simulink model "towTest"  (R2020a)
settings: Solver=FixedStepAuto  StartTime=0.0  StopTime=inf  RelTol=1e-3  EnableMultiTasking=on
undefined symbols (not defined in the file or in its folder): IO397
libraries: slrtlib x5, speedgoatlib_fpga_quadrature x2, dspsigops x2, speedgoatlib_fpga_dio x1, speedgoatlib_fpga_analog_io x1, dspfdesign x1, speedgoatlib_fpga x1, powerlib_meascontrol x1
settings Model: SimulationMode=external  Creator=MAE-VermillionLab  LastModifiedBy=ViconLab
settings SolverCC: ConcurrentTasks=on  AutoInsertRateTranBlk=on
settings DataIOCC: SaveFormat=StructureWithTime
settings OptimizationCC: BlockReduction=off  OptimizeBlockIOStorage=off
settings HardwareCC: ProdBitPerPointer=32  ProdBitPerSizeT=32  ProdBitPerPtrDiffT=32  ProdLargestAtomicFloat=None  ProdWordSize=32  ProdLongLongMode=on  ProdHWDeviceType=Generic->32-bit x86 compatible
settings RTWCC: Description=Simulink Real-Time  SystemTargetFile=slrt.tlc  TemplateMakefile=slrt_default_tmf  CodeExecutionProfiling=on  RTWCompilerOptimization=on
settings SimulinkRealTimeCC: SupportVariableSizeSignals=on  RL32LogTETModifier=off  xPCConcurrentTasks=on

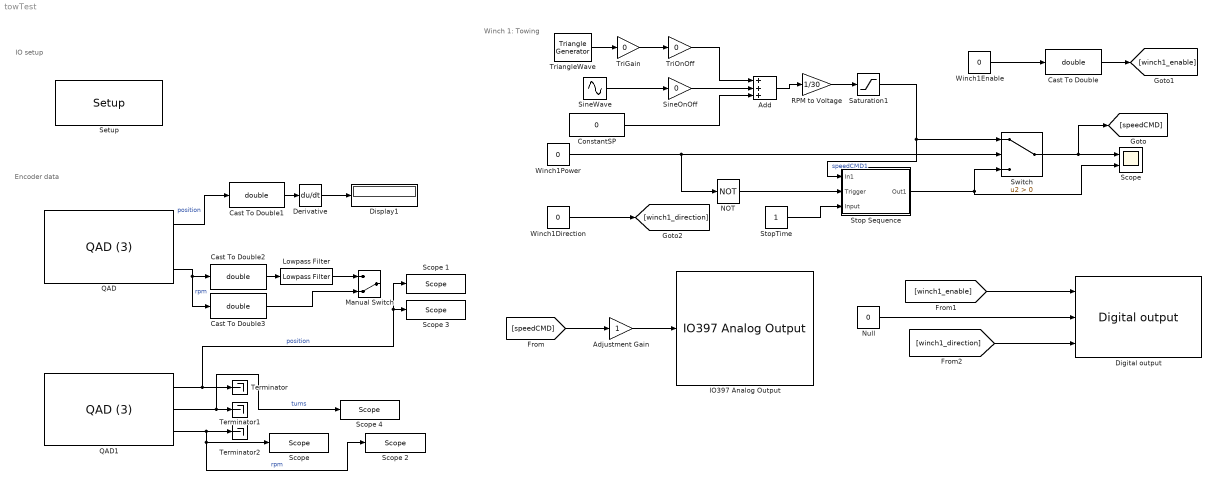
== system towTest ==
  note: Winch 1: Towing
  note: Encoder data
  note: IO setup
  Add : Sum  Inputs=+++
  Adjustment Gain : Gain
  Cast To Double{,1..3} (4 alike) : DataTypeConversion  OutDataTypeStr=double
  ConstantSP : Constant  Value=0
  Derivative : Derivative
  Digital output : speedgoatlib_fpga_dio/Digital output  id=1  chan=[1:3]  init=[0]  reset=[0]  vectorizeInput=off  ts=Ts  pciSlot=-1  board=IO397-50k
      settings: SourceProductName=Simulink Real-Time: Speedgoat I/O Driver Library
  Display1 : Display
  IO397 Analog Output : speedgoatlib_fpga_analog_io/IO397 Analog Output  id=1  chan=1  initVal=0  resetVal=0  ts=0.001  pciSlot=-1  board=IO397-50k  span=+5 V
      settings: SourceProductName=Simulink Real-Time: Speedgoat I/O Driver Library
  Lowpass Filter : dspfdesign/Lowpass Filter  FilterType=FIR  DesignForMinimumOrder=on  FilterOrder=50  PassbandFrequency=100  StopbandFrequency=1.2e3  PassbandRipple=0.1  StopbandAttenuation=80  InheritSampleRate=off  SampleRate=44100  SimulateUsing=Interpreted execution  roundingMode=Floor  coeffsDataTypeStr=fixdt(1,16)
  Manual Switch : ManualSwitch  CurrentSetting=0
  NOT : Logic  Operator=NOT  IconShape=distinctive  AllPortsSameDT=off  OutDataTypeStr=boolean
  Null : Constant  Value=0
  QAD : speedgoatlib_fpga_quadrature/QAD (3)  id=1  board=IO397-50k  chan=[1]  resetOnStart=on  ts=Ts  pciSlot=-1  operatingMode=Quadrature decoder  indexControlMode=Ignore index  resolution=1x  stepsPerRevolution=[1800]  latchMode=Software latch  interpolatePosition=off  invertAB=off  showClearPositionInput=off  showClearIndexFoundInput=off  showPositionOutput=on  showTurnOutput=on  showSpeedOutput=on  showDirectionOutput=off  showIndexFoundOutput=off
      settings: SourceProductName=Simulink Real-Time: Speedgoat I/O Driver Library
  QAD1 : speedgoatlib_fpga_quadrature/QAD (3)  id=1  board=IO397-50k  chan=[2]  resetOnStart=on  ts=Ts  pciSlot=-1  operatingMode=Quadrature decoder  indexControlMode=Ignore index  resolution=2x  stepsPerRevolution=1800  latchMode=Disabled  interpolatePosition=off  invertAB=off  showClearPositionInput=off  showClearIndexFoundInput=off  showPositionOutput=on  showTurnOutput=on  showSpeedOutput=on  showDirectionOutput=off  showIndexFoundOutput=off
      settings: SourceProductName=Simulink Real-Time: Speedgoat I/O Driver Library
  RPM to Voltage : Gain  Gain=1/30
  Saturation1 : Saturate  UpperLimit=5  LowerLimit=0
  Scope : Scope  NumInputPorts=2
  "Scope " : slrtlib/Displays and Logging/Scope   scopeno=1  scopetype=Target  autostart=on  viewmode=Numerical  formatstr='%15.6f'  grid=on  ylimits=[0,0]  nosamples=2000  noprepostsamples=0  interleave=1  triggermode=FreeRun  triggersignal=1  trigsignalfromport=off  triggerlevel=0.0  triggerslope=Either  triggerscope=1  triggersample=0  filename=data.dat  mode=Lazy  writesize=512  autorestart=off  dynamicfilemode=off  maxwritefilesize=512*1024^2
  Scope 1 : slrtlib/Displays and Logging/Scope   scopeno=2  scopetype=Target  autostart=on  viewmode=Numerical  formatstr='%15.6f'  grid=on  ylimits=[0,0]  nosamples=1000  noprepostsamples=0  interleave=1  triggermode=FreeRun  triggersignal=1  trigsignalfromport=off  triggerlevel=0.0  triggerslope=Either  triggerscope=1  triggersample=0  filename=data.dat  mode=Lazy  writesize=512  autorestart=off  dynamicfilemode=off  maxwritefilesize=512*1024^2
  Scope 2 : slrtlib/Displays and Logging/Scope   scopeno=3  scopetype=Target  autostart=on  viewmode=Graphical sliding  formatstr='%15.6f'  grid=on  ylimits=[0,5000]  nosamples=1000  noprepostsamples=0  interleave=1  triggermode=FreeRun  triggersignal=1  trigsignalfromport=off  triggerlevel=0.0  triggerslope=Either  triggerscope=1  triggersample=0  filename=data.dat  mode=Lazy  writesize=512  autorestart=off  dynamicfilemode=off  maxwritefilesize=512*1024^2
  Scope 3 : slrtlib/Displays and Logging/Scope   scopeno=4  scopetype=Target  autostart=on  viewmode=Graphical sliding  formatstr='%15.6f'  grid=on  ylimits=[0,4000]  nosamples=1000  noprepostsamples=0  interleave=1  triggermode=FreeRun  triggersignal=1  trigsignalfromport=off  triggerlevel=0.0  triggerslope=Either  triggerscope=1  triggersample=0  filename=data.dat  mode=Lazy  writesize=512  autorestart=off  dynamicfilemode=off  maxwritefilesize=512*1024^2
  Scope 4 : slrtlib/Displays and Logging/Scope   scopeno=5  scopetype=Target  autostart=on  viewmode=Numerical  formatstr='%15.6f'  grid=on  ylimits=[0,0]  nosamples=1000  noprepostsamples=0  interleave=1  triggermode=FreeRun  triggersignal=1  trigsignalfromport=off  triggerlevel=0.0  triggerslope=Either  triggerscope=1  triggersample=0  filename=data.dat  mode=Lazy  writesize=512  autorestart=off  dynamicfilemode=off  maxwritefilesize=512*1024^2
  Setup : speedgoatlib_fpga/Setup/Setup  board=IO397-50k  id=1  device_id=1  frontIO=None  rearIO=None  bitstreamFile=speedgoat_IO397_50k_CI_02113  rev=1.0  timestamp_string=21/04/20 11:41:53  fpgaFreq=75 MHz  fpgaTick=13.33 ns  ProgSpiFlash=off  ProgBPIFlash=off  pciSlot=-1  PullRPort0=pull-up 3.3V  VioPort0=3.3V  PullRPort1=pull-up 3.3V  VioPort1=3.3V  PullRPort2=pull-up 3.3V  VioPort2=3.3V  PullRPort3=pull-up 3.3V  VioPort3=3.3V  PullRPort4=pull-up 3.3V  VioPort4=3.3V  PullRPort5=pull-up 3.3V  VioPort5=3.3V  PullRPort6=pull-up 3.3V  VioPort6=3.3V  PullRPort15=pull-up 3.3V  PullRPort31=pull-up 3.3V  PullRPort47=pull-up 3.3V  PullRPort63=pull-up 3.3V
      settings: SourceProductName=Simulink Real-Time: Speedgoat Library
  SineOnOff : Gain  Gain=0
  SineWave : Sin  Amplitude=0  Frequency=6.2832  SampleTime=0
  "Stop Sequence " : Subsystem  TreatAsAtomicUnit=on
  StopTime : Constant
  Switch : Switch  Criteria=u2 > Threshold
  Terminator : Terminator
  Terminator1 : Terminator
  Terminator2 : Terminator
  TriGain : Gain  Gain=0
  TriOnOff : Gain  Gain=0
  TriangleWave : powerlib_meascontrol/Pulse & Signal Generators/Triangle Generator  Freq=1  Phase=90  Ts=0
  Winch1Direction : Constant  Value=0
  Winch1Enable : Constant  Value=0
  Winch1Power : Constant  Value=0
  wires:
  QAD/1 -> Cast To Double1/1  "position"
  QAD/3 -> Cast To Double3/1, Cast To Double2/1  "rpm"
  QAD1/1 -> Scope 3/1, Scope 1/1, Terminator/1  "position"
  "Stop Sequence "/1(Out1) -> Scope/2, Switch/3
  Switch/1 -> [speedCMD], Scope/1
  Winch1Power/1 -> NOT/1, Switch/2
  NOT/1 -> "Stop Sequence "/2(Trigger)
  Saturation1/1 -> "Stop Sequence "/1(In1), Switch/1  "speedCMD1"
  [speedCMD] -> Adjustment Gain/1
  Adjustment Gain/1 -> IO397 Analog Output/1
  [winch1_enable] -> Digital output/1
  Winch1Direction/1 -> [winch1_direction]
  Cast To Double/1 -> [winch1_enable]
  Winch1Enable/1 -> Cast To Double/1
  Derivative/1 -> Display1/1
  Cast To Double1/1 -> Derivative/1
  Cast To Double2/1 -> Lowpass Filter/1
  Lowpass Filter/1 -> Manual Switch/1
  Cast To Double3/1 -> Manual Switch/2
  QAD1/2 -> Scope 4/1, Terminator1/1  "turns"
  QAD1/3 -> Scope 2/1, "Scope "/1, Terminator2/1  "rpm"
  ConstantSP/1 -> Add/3
  Add/1 -> RPM to Voltage/1
  SineOnOff/1 -> Add/2
  [winch1_direction] -> Digital output/3
  Null/1 -> Digital output/2
  TriOnOff/1 -> Add/1
  RPM to Voltage/1 -> Saturation1/1
  TriangleWave/1 -> TriGain/1
  TriGain/1 -> TriOnOff/1
  SineWave/1 -> SineOnOff/1
  StopTime/1 -> "Stop Sequence "/3(Input)

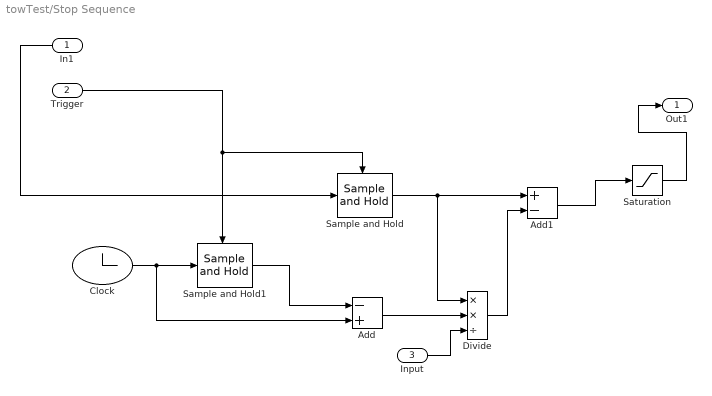
== system towTest/Stop Sequence  ==
  In1 : Inport
  Trigger : Inport  Port=2
  Input : Inport  Port=3
  Add : Sum  Inputs=-+
  Add1 : Sum  Inputs=+-
  Clock : Clock
  Divide : Product  Inputs=**/
  Sample and Hold : dspsigops/Sample and Hold  trig=Rising edge  initCond=0  latchinput=off
  Sample and Hold1 : dspsigops/Sample and Hold  trig=Rising edge  initCond=0  latchinput=off
  Saturation : Saturate  UpperLimit=5  LowerLimit=0
  Out1 : Outport
  wires:
  Trigger/1 -> Sample and Hold1/Trigger, Sample and Hold/Trigger
  Add/1 -> Divide/2
  In1/1 -> Sample and Hold/1
  Divide/1 -> Add1/2
  Sample and Hold/1 -> Divide/1, Add1/1
  Sample and Hold1/1 -> Add/1
  Clock/1 -> Add/2, Sample and Hold1/1
  Add1/1 -> Saturation/1
  Saturation/1 -> Out1/1
  Input/1 -> Divide/3
